simulink model "sensor_board_board_to_MCU"  (R2022a)
settings: Solver=FixedStepAuto  StartTime=0.0  StopTime=Inf  RelTol=1e-3  EnableMultiTasking=on
libraries: c2802xlib x4, canmsglib x2, c280xlib x2, c2837xDlib x1
settings Model: ExtModeTrigDuration=8  Creator=Joe Wild  LastModifiedBy=Joe Wild
settings OptimizationCC: DefaultUnderspecifiedDataType=single  EnhancedBackFolding=on  PassReuseOutputArgsAs=Individual arguments  MaxStackSize=1024  OptimizeBlockOrder=speed  DifferentSizesBufferReuse=on  OptimizationCustomize=off  DenormalBehavior=FlushToZero  EfficientTunableParamExpr=on
settings DebuggingCC: ParameterTunabilityLossMsg=error
settings HardwareCC: ProdBitPerChar=16  ProdBitPerInt=16  ProdBitPerPointer=32  ProdBitPerSizeT=32  ProdBitPerPtrDiffT=32  ProdLargestAtomicInteger=Integer  ProdLargestAtomicFloat=None  ProdWordSize=16  ProdLongLongMode=on  ProdHWDeviceType=Texas Instruments->C2000
settings SFSimCC: MATLABDynamicMemAlloc=off
settings RTWCC: SystemTargetFile=ert.tlc  HardwareBoard=TI Delfino F28379D LaunchPad  TemplateMakefile=ert_default_tmf  Toolchain=Texas Instruments Code Composer Studio (C2000)
settings CodeAppCC: ForceParamTrailComments=on  IgnoreCustomStorageClasses=off  OperatorAnnotations=on  SimulinkDataObjDesc=on  SFDataObjDesc=on  InsertBlockDesc=on
settings ERTTargetCC: CodeReplacementLibrary=TI C28x  ExtModeTransport=4  ExtModeStaticAlloc=on  ExtModeMexFile=ext_xcp  ExtModeIntrfLevel=Level2 - Open

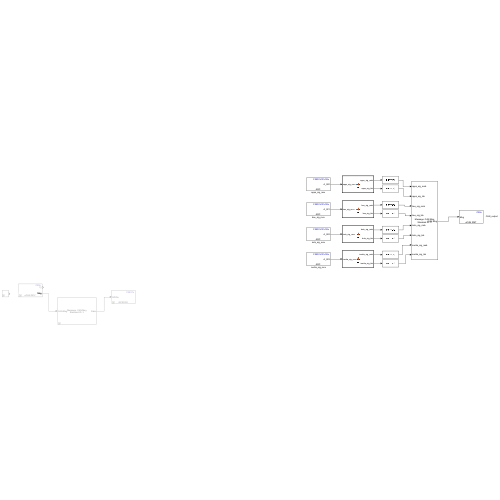
[thumbnail: Simulink's stored preview of the top-level diagram]
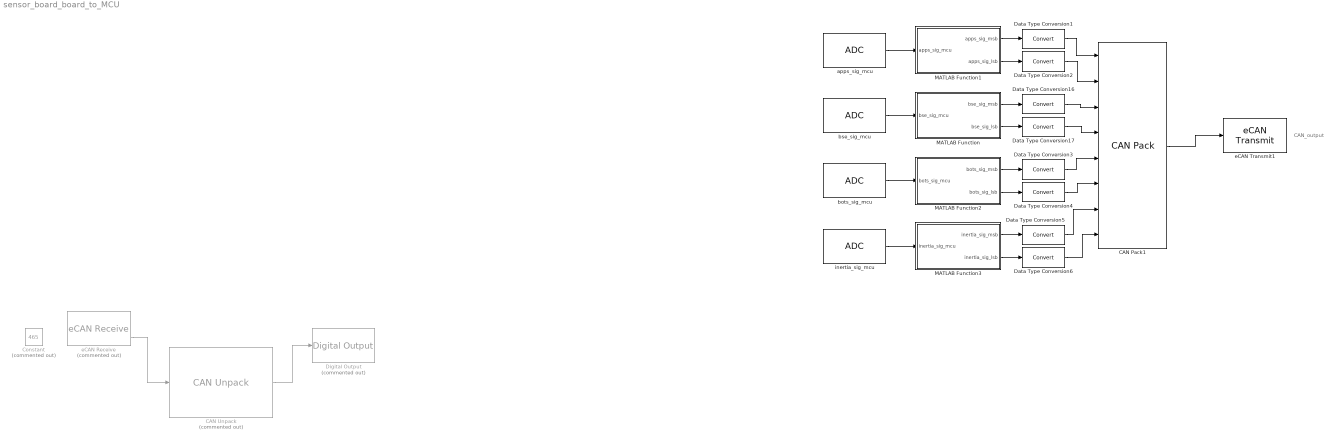
== system sensor_board_board_to_MCU ==
  note: CAN_output
  CAN Pack1 : canmsglib/CAN Pack  MsgList=(none)  MsgName=CAN Msg  MsgIDType=Standard (11-bit identifier)  MsgIdentifier=0  MsgLength=8  Remote=off  ApplyMinMax=off  BusOutput=off  SignalInfo={ 'apps_sig_msb', '0', '8', 'LE', 'unsigned', 'Standard', '0', '1', '0', '-Inf', 'Inf'; 'apps_sig_lsb', '8', '8', 'LE', 'unsigned', 'Standard', '0', '1', '0', '-Inf', 'Inf'; 'bse_sig_msb', '16', '8', 'LE', 'signed', 'Standard', '0', '1', '0', '-Inf', 'Inf'; 'bse_sig_lsb', '24', '8', 'LE', 'signed', 'Standard', '0', '1', '0', '-Inf', 'Inf'; 'bots_sig_msb', '32', '8', 'LE', 'signed', 'Standard', '0', '1', '0', '-Inf', 'Inf'; 'bots_sig_lsb', '40', '8', 'LE', 'signed', 'Standard', '0', '1', '0', '-Inf', 'Inf'; 'inertia_sig_msb', '48', '8', 'LE', 'signed', 'Standard', '0', '1', '0', '-Inf', 'Inf'; 'inertia_sig_lsb', '56', '8', 'LE', 'signed', 'Standard', '0', '1', '0', '-Inf', 'Inf' }
      settings: SourceProductBaseCode=ME,XP,VN  DataFormat=manually specified signals
  CAN Unpack : canmsglib/CAN Unpack  Commented=on  MsgList=(none)  MsgName=CAN Msg  MsgIDType=Standard (11-bit identifier)  MsgIdentifier=3  MsgLength=1  SignalInfo={}  IDPort=off  TimestampPort=off  ErrorPort=off  RemotePort=off  LengthPort=off  StatusPort=off  ApplyMinMax=off
      settings: SourceProductBaseCode=XP,ME,VN  DataFormat=raw data
  Constant : Constant  Commented=on  Value=465
  Data Type Conversion{1..6,16..17} (8 alike) : DataTypeConversion  SaturateOnIntegerOverflow=off  RndMeth=Floor
  Digital Output : c2837xDlib/Digital Output  Commented=on  GPIO_Number=GPIO104~GPIO111  GPIO_Bit0=off  GPIO_BIT0_Toggle=off  GPIO_Bit1=off  GPIO_BIT1_Toggle=off  GPIO_Bit2=off  GPIO_BIT2_Toggle=off  GPIO_Bit3=off  GPIO_BIT3_Toggle=off  GPIO_Bit4=off  GPIO_BIT4_Toggle=off  GPIO_Bit5=off  GPIO_BIT5_Toggle=off  GPIO_Bit6=off  GPIO_BIT6_Toggle=off  GPIO_Bit7=on  GPIO_BIT7_Toggle=on
      settings: SourceProductBaseCode=TIC2000
  MATLAB Function : MATLAB Function  TreatAsAtomicUnit=on
  MATLAB Function1 : MATLAB Function  TreatAsAtomicUnit=on
  MATLAB Function2 : MATLAB Function  TreatAsAtomicUnit=on
  MATLAB Function3 : MATLAB Function  TreatAsAtomicUnit=on
  apps_sig_mcu : c2802xlib/ADC  blkParamProc=C2000_Type4  ADCModule=A  samplingMode=Single sample mode  ADCResolution=12-bit (Single-ended input)  useSOC1=SOC0  useSOC2=SOC0_SOC1  SOCAcquisitionWindow=60  SOCTriggerSource=Software  SOCInterruptTrigger=No ADCINT  Ts=0.001  dType=uint16  postInterrupt=off  interruptSel=ADCINT1  ADCINTContinuous=on  endma=off  chdma=1  conv1=ADCINA0  conv2=ADCINA0 and ADCINB0  conv1_Type4=ADCIN0  conv2_Type4=ADCIN0 and ADCIN1
  bots_sig_mcu : c2802xlib/ADC  blkParamProc=C2000_Type4  ADCModule=A  samplingMode=Single sample mode  ADCResolution=12-bit (Single-ended input)  useSOC1=SOC2  useSOC2=SOC0_SOC1  SOCAcquisitionWindow=60  SOCTriggerSource=Software  SOCInterruptTrigger=No ADCINT  Ts=0.001  dType=uint16  postInterrupt=off  interruptSel=ADCINT1  ADCINTContinuous=on  endma=off  chdma=1  conv1=ADCINA0  conv2=ADCINA0 and ADCINB0  conv1_Type4=ADCIN2  conv2_Type4=ADCIN0 and ADCIN1
  bse_sig_mcu : c2802xlib/ADC  blkParamProc=C2000_Type4  ADCModule=A  samplingMode=Single sample mode  ADCResolution=12-bit (Single-ended input)  useSOC1=SOC1  useSOC2=SOC0_SOC1  SOCAcquisitionWindow=60  SOCTriggerSource=Software  SOCInterruptTrigger=No ADCINT  Ts=0.001  dType=uint16  postInterrupt=off  interruptSel=ADCINT1  ADCINTContinuous=on  endma=off  chdma=1  conv1=ADCINA0  conv2=ADCINA0 and ADCINB0  conv1_Type4=ADCIN1  conv2_Type4=ADCIN0 and ADCIN1
  eCAN Receive : c280xlib/eCAN Receive  Commented=on  chipFamily=C280x  useModule=eCAN_B  mailboxNo=1  messageID=3  messageType=Standard (11-bit identifier)  enableAcceptanceFiltering=off  messageIDMask=0  sampleTime=1  dataType=CAN_MESSAGE_TYPE  outputAction=Output last received values  initValue=0  outputMessageID=off  outputMessageLength=off  outputMessageTimeStamp=off  postInterrupt=off  interruptLine=0
      settings: SourceProductBaseCode=TIC2000
  eCAN Transmit1 : c280xlib/eCAN Transmit  chipFamily=C280x  useModule=eCAN_B  mailboxNo=2  messageID=2  messageType=Standard (11-bit identifier)  enableBlockingMode=off  postInterrupt=off  interruptLine=0
      settings: SourceProductBaseCode=TIC2000
  inertia_sig_mcu : c2802xlib/ADC  blkParamProc=C2000_Type4  ADCModule=A  samplingMode=Single sample mode  ADCResolution=12-bit (Single-ended input)  useSOC1=SOC3  useSOC2=SOC0_SOC1  SOCAcquisitionWindow=60  SOCTriggerSource=Software  SOCInterruptTrigger=No ADCINT  Ts=0.001  dType=uint16  postInterrupt=off  interruptSel=ADCINT1  ADCINTContinuous=on  endma=off  chdma=1  conv1=ADCINA0  conv2=ADCINA0 and ADCINB0  conv1_Type4=ADCIN3  conv2_Type4=ADCIN0 and ADCIN1
  wires:
  eCAN Receive/2 -> CAN Unpack/1
  CAN Unpack/1 -> Digital Output/1
  bse_sig_mcu/1 -> MATLAB Function/1(bse_sig_mcu)
  MATLAB Function/2(bse_sig_lsb) -> Data Type Conversion17/1
  MATLAB Function/1(bse_sig_msb) -> Data Type Conversion16/1
  Data Type Conversion17/1 -> CAN Pack1/4
  Data Type Conversion16/1 -> CAN Pack1/3
  apps_sig_mcu/1 -> MATLAB Function1/1(apps_sig_mcu)
  Data Type Conversion1/1 -> CAN Pack1/1
  CAN Pack1/1 -> eCAN Transmit1/1
  MATLAB Function1/1(apps_sig_msb) -> Data Type Conversion1/1
  Data Type Conversion2/1 -> CAN Pack1/2
  MATLAB Function1/2(apps_sig_lsb) -> Data Type Conversion2/1
  bots_sig_mcu/1 -> MATLAB Function2/1(bots_sig_mcu)
  Data Type Conversion3/1 -> CAN Pack1/5
  MATLAB Function2/1(bots_sig_msb) -> Data Type Conversion3/1
  Data Type Conversion4/1 -> CAN Pack1/6
  MATLAB Function2/2(bots_sig_lsb) -> Data Type Conversion4/1
  inertia_sig_mcu/1 -> MATLAB Function3/1(inertia_sig_mcu)
  Data Type Conversion5/1 -> CAN Pack1/7
  MATLAB Function3/1(inertia_sig_msb) -> Data Type Conversion5/1
  Data Type Conversion6/1 -> CAN Pack1/8
  MATLAB Function3/2(inertia_sig_lsb) -> Data Type Conversion6/1

== matlab function sensor_board_board_to_MCU/MATLAB Function1 ==
  data: apps_sig_mcu input; apps_sig_msb output; apps_sig_lsb output
function [apps_sig_msb, apps_sig_lsb]= fcn(apps_sig_mcu)
%#codegen

%Note: ADC output is in uint16. Performing operations with this produces an integer, so it is first converted to a double to allow for decimals.
apps_sig_msb = floor(double(apps_sig_mcu) / 256); %Every time the line below loops, this increments by 1. floor = round down.
apps_sig_lsb = rem(apps_sig_mcu,256); %Counts up to 256 then loops back down to zero. rem = remainder

== matlab function sensor_board_board_to_MCU/MATLAB Function ==
  data: bse_sig_mcu input; bse_sig_msb output; bse_sig_lsb output
function [bse_sig_msb, bse_sig_lsb]= fcn(bse_sig_mcu)
%#codegen

%Note: ADC output is in uint16. Performing operations with this produces an integer, so it is first converted to a double to allow for decimals.
bse_sig_msb = floor(double(bse_sig_mcu) / 256); %Every time the line below loops, this increments by 1. floor = round down.
bse_sig_lsb = rem(bse_sig_mcu,256); %Counts up to 256 then loops back down to zero. rem = remainder

== matlab function sensor_board_board_to_MCU/MATLAB Function2 ==
  data: bots_sig_mcu input; bots_sig_msb output; bots_sig_lsb output
function [bots_sig_msb, bots_sig_lsb]= fcn(bots_sig_mcu)
%#codegen

%Note: ADC output is in uint16. Performing operations with this produces an integer, so it is first converted to a double to allow for decimals.
bots_sig_msb = floor(double(bots_sig_mcu) / 256); %Every time the line below loops, this increments by 1. floor = round down.
bots_sig_lsb = rem(bots_sig_mcu,256); %Counts up to 256 then loops back down to zero. rem = remainder

== matlab function sensor_board_board_to_MCU/MATLAB Function3 ==
  data: inertia_sig_mcu input; inertia_sig_msb output; inertia_sig_lsb output
function [inertia_sig_msb, inertia_sig_lsb]= fcn(inertia_sig_mcu)
%#codegen

%Note: ADC output is in uint16. Performing operations with this produces an integer, so it is first converted to a double to allow for decimals.
inertia_sig_msb = floor(double(inertia_sig_mcu) / 256); %Every time the line below loops, this increments by 1. floor = round down.
inertia_sig_lsb = rem(inertia_sig_mcu,256); %Counts up to 256 then loops back down to zero. rem = remainder
